simulink model "AGTF30SysSS_PExPIn"  (R2021b)
settings: Solver=FixedStepDiscrete  StartTime=0.0  StopTime=0; %MWS.In.Ts  FixedStep=1  RelTol=1e-3  EnableMultiTasking=on
values from neighbouring files (symbols this model uses):
  MWS = setup_initialize(MWS,startPt,SSsolverSP)    [Setup_Simulation.m]    (also in run_AGTF30e_script.m = Setup_Simulation(inputMethod,MWS.In,filename,Mdl,SSsolverSP,)
libraries: simulink x66, Lib_Solve_SSNRSolverJC_TMATS x1
(part 1 of 2)
settings Model: Creator=jwchapm2  LastModifiedBy=jlkratz
settings SolverCC: AlgebraicLoopSolver=TrustRegion
settings DataIOCC: LimitDataPoints=on  SaveFormat=Array  ReturnWorkspaceOutputs=off
settings OptimizationCC: LifeSpan=inf
settings DebuggingCC: SFUnexpectedBacktrackingDiag=warning  SFNoUnconditionalDefaultTransitionDiag=warning  SFExecutionAtInitializationDiag=none  SFMachineParentedDataDiag=warning  ArithmeticOperatorsInVariantConditions=warning
settings HardwareCC: ProdBitPerPointer=32  ProdBitPerSizeT=32  ProdBitPerPtrDiffT=32  ProdLargestAtomicFloat=None  ProdIntDivRoundTo=Undefined  ProdEndianess=Unspecified  ProdWordSize=32  ProdHWDeviceType=32-bit Generic
settings ModelReferenceCC: PropagateSignalLabelsOutOfModel=off
settings SFSimCC: SimUseLocalCustomCode=off  CustomCodeUndefinedFunction=UseInterfaceOnly
settings RTWCC: RTWUseLocalCustomCode=off
settings CodeAppCC: StateflowObjectComments=on
settings GRTTargetCC: TargetLangStandard=C89/C90 (ANSI)
settings ConfigComp: CovMetricSettings=dw  CovSaveCumulativeToWorkspaceVar=on  CovSaveSingleToWorkspaceVar=on  CovExternalEMLEnable=off

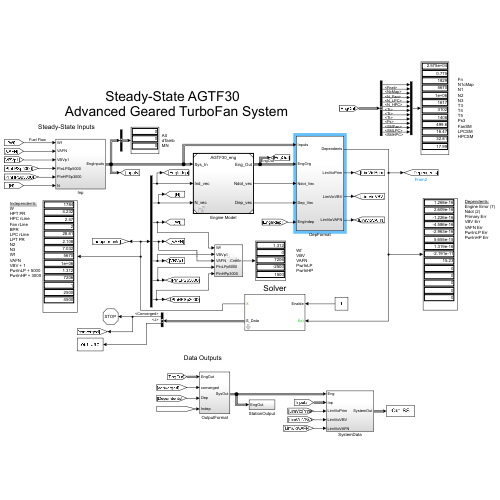
[thumbnail: Simulink's stored preview of the top-level diagram]
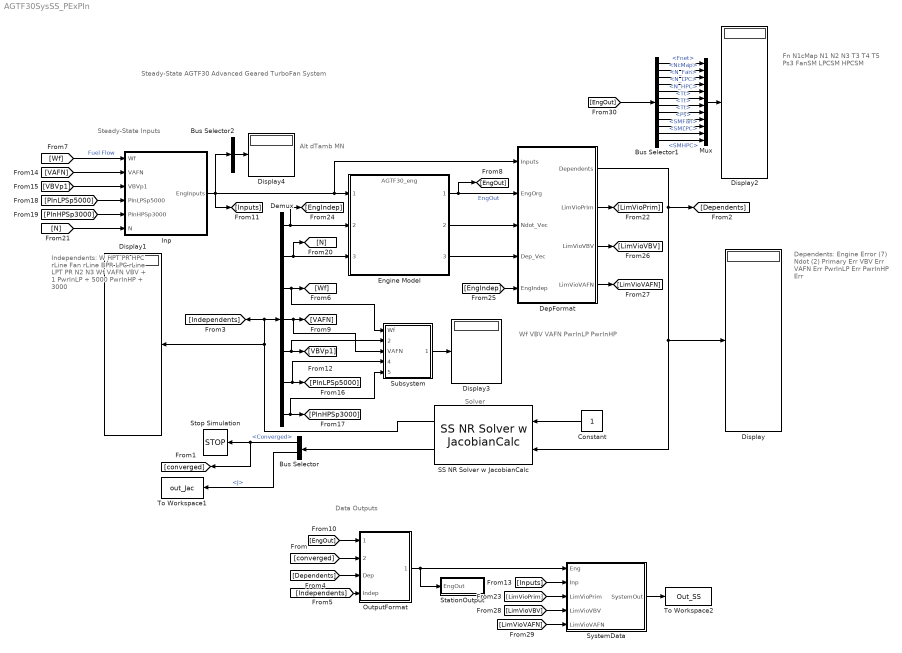
== system AGTF30SysSS_PExPIn ==
  note: Independents:
      | W
      | HPT PR
      | HPC rLine
      | Fan rLine
      | BPR
      | LPC rLine
      | LPT PR
      | N2
      | N3
      | Wf
      | VAFN
      | VBV + 1
      | PwrInLP + 5000
      | PwrInHP + 3000
  note: Dependents:
      | Engine Error (7)
      | Ndot (2)
      | Primary Err
      | VBV Err
      | VAFN Err
      | PwrInLP Err
      | PwrInHP Err
  note: Alt
      | dTamb
      | MN
  note: Wf
      | VBV
      | VAFN
      | PwrInLP
      | PwrInHP
  note: Fn
      | N1cMap
      | N1
      | N2
      | N3
      | T3
      | T4
      | T5
      | Ps3
      | FanSM
      | LPCSM
      | HPCSM
  note: Solver
  note: Steady-State Inputs
  note: Data Outputs
  note: Steady-State AGTF30
      | Advanced Geared TurboFan System
  Bus Selector : BusSelector  OutputSignals=Converged,J
  Bus Selector1 : BusSelector  OutputSignals=Perf.Fnet,Data.FAN_Data.NcMap,Shaft.N_Fan,Shaft.N_LPC,Shaft.N_HPC,S36.Tt,S4.Tt,S5.Tt,S36.Ps,SM.SMFan,SM.SMLPC,SM.SMHPC
  Bus Selector2 : BusSelector  OutputSignals=Altitude,dTamb,MN  OutputAsBus=on
  Constant : Constant
  Demux : Demux  Outputs=[7 2 1 1 1 1 1]
  DepFormat : Subsystem
  Display{,1..4} (5 alike) : Display
  Engine Model : ModelReference  ModelNameDialog=AGTF30_eng.mdl  SimulationMode=Normal  ModelReferenceVersion=14.20
  Inp : Subsystem
  Mux : Mux  Inputs=12
  OutputFormat : Subsystem
  SS NR Solver w JacobianCalc : Lib_Solve_SSNRSolverJC_TMATS/SS NR Solver w JacobianCalc  SJac_Per_M=MWS.Init.Solver.SS.JPer  SNR_IC_M=MWS.Init.Solver.SS.IC  SNR_DX_M=MWS.Init.Solver.SS.dX  SNR_Mx_M=1000000  SNR_Mn_M=0.000001  SJacobianAttempts_M=MWS.Init.Solver.SS.NRA  Cond_Limits_M=MWS.Init.Solver.SS.Lim
  StationOutput : Subsystem
  Stop Simulation : Stop
  Subsystem : Subsystem
  SystemData : Subsystem
  To Workspace1 : ToWorkspace  VariableName=out_Jac  SaveFormat=Timeseries  SampleTime=-1
      settings: MaxDataPoints=1
  To Workspace2 : ToWorkspace  VariableName=Out_SS  SaveFormat=Timeseries  SampleTime=-1
      settings: MaxDataPoints=1
  wires:
  Demux/2 -> [N], Engine Model/3
  Demux/1 -> [EngIndep], Engine Model/2
  Constant/1 -> SS NR Solver w JacobianCalc/1
  SS NR Solver w JacobianCalc/2 -> Bus Selector/1
  Bus Selector/1 -> Stop Simulation/1, [converged]  "<Converged>"
  Engine Model/1 -> [EngOut], DepFormat/2(EngOrg)  "EngOut"
  SS NR Solver w JacobianCalc/1 -> Display1/1, [Independents], Demux/1
  Demux/3 -> Subsystem/1(Wf), [Wf]
  DepFormat/1(Dependents) -> SS NR Solver w JacobianCalc/2, Display/1, [Dependents]
  Engine Model/2 -> DepFormat/3(Ndot_Vec)
  [converged] -> OutputFormat/2(converged)
  [Dependents] -> OutputFormat/3(Dep)
  [Independents] -> OutputFormat/4(Indep)
  [EngOut] -> OutputFormat/1(EngOut)
  Inp/1(EngInputs) -> Bus Selector2/1, [Inputs], DepFormat/1(Inputs), Engine Model/1
  [Wf] -> Inp/1(Wf)  "Fuel Flow"
  OutputFormat/1(SysOut) -> StationOutput/1(EngOut), SystemData/1(Eng)
  SystemData/1(SystemOut) -> To Workspace2/1
  [Inputs] -> SystemData/2(Inp)
  Engine Model/3 -> DepFormat/4(Dep_Vec)
  [VAFN] -> Inp/2(VAFN)
  Demux/4 -> Subsystem/3(VAFN), [VAFN]
  [VBVp1] -> Inp/3(VBVp1)
  Demux/6 -> Subsystem/4(PInLPp5000), [PInLPSp5000]
  Demux/7 -> [PInHPSp3000], Subsystem/5(PInHPp3000)
  [PInHPSp3000] -> Inp/5(PInHPSp3000)
  [PInLPSp5000] -> Inp/4(PInLPSp5000)
  [N] -> Inp/6(N)
  DepFormat/2(LimVioPrim) -> [LimVioPrim]
  [LimVioPrim] -> SystemData/3(LimVioPrim)
  [EngIndep] -> DepFormat/5(EngIndep)
  DepFormat/3(LimVioVBV) -> [LimVioVBV]
  DepFormat/4(LimVioVAFN) -> [LimVioVAFN]
  [LimVioVBV] -> SystemData/4(LimVioVBV)
  [LimVioVAFN] -> SystemData/5(LimVioVAFN)
  [EngOut] -> Bus Selector1/1
  Mux/1 -> Display2/1
  Subsystem/1(CntrlIn) -> Display3/1
  Demux/5 -> [VBVp1], Subsystem/2(VBVp1)
  Bus Selector2/1 -> Display4/1
  Bus Selector1/1 -> Mux/1  "<Fnet>"
  Bus Selector1/3 -> Mux/3  "<N_Fan>"
  Bus Selector1/5 -> Mux/5  "<N_HPC>"
  Bus Selector1/4 -> Mux/4  "<N_LPC>"
  Bus Selector1/6 -> Mux/6  "<Tt>"
  Bus Selector1/7 -> Mux/7  "<Tt>"
  Bus Selector1/8 -> Mux/8  "<Tt>"
  Bus Selector1/10 -> Mux/10  "<SMFan>"
  Bus Selector1/9 -> Mux/9  "<Ps>"
  Bus Selector1/11 -> Mux/11  "<SMLPC>"
  Bus Selector1/12 -> Mux/12  "<SMHPC>"
  Bus Selector/2 -> To Workspace1/1  "<J>"
  Bus Selector1/2 -> Mux/2  "<NcMap>"

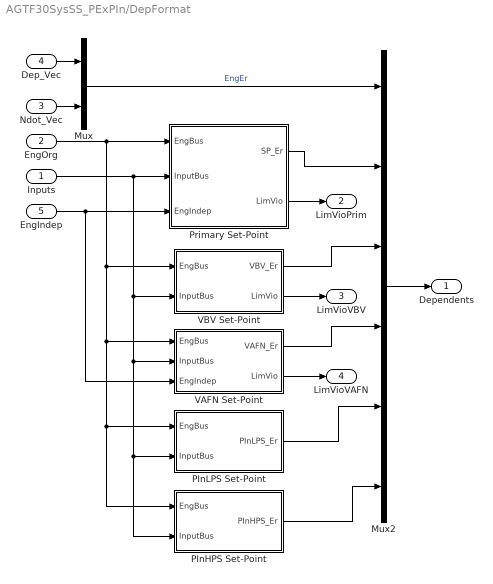
== system AGTF30SysSS_PExPIn/DepFormat ==
  Inputs : Inport
  EngOrg : Inport  Port=2
  Ndot_Vec : Inport  Port=3
  Dep_Vec : Inport  Port=4
  EngIndep : Inport  Port=5
  Mux : Mux  Inputs=2
  Mux2 : Mux  Inputs=6
  PInHPS Set-Point : Subsystem
  PInLPS Set-Point : Subsystem
  Primary Set-Point : Subsystem
  VAFN Set-Point : Subsystem
  VBV Set-Point : Subsystem
  Dependents : Outport
  LimVioPrim : Outport  Port=2
  LimVioVBV : Outport  Port=3
  LimVioVAFN : Outport  Port=4
  wires:
  Ndot_Vec/1 -> Mux/2
  Mux/1 -> Mux2/1  "EngEr"
  Mux2/1 -> Dependents/1
  Dep_Vec/1 -> Mux/1
  EngOrg/1 -> PInHPS Set-Point/1(EngBus), PInLPS Set-Point/1(EngBus), VAFN Set-Point/1(EngBus), VBV Set-Point/1(EngBus), Primary Set-Point/1(EngBus)
  Inputs/1 -> Primary Set-Point/2(InputBus), PInHPS Set-Point/2(InputBus), PInLPS Set-Point/2(InputBus), VAFN Set-Point/2(InputBus), VBV Set-Point/2(InputBus)
  Primary Set-Point/1(SP_Er) -> Mux2/2
  VBV Set-Point/1(VBV_Er) -> Mux2/3
  VAFN Set-Point/1(VAFN_Er) -> Mux2/4
  PInLPS Set-Point/1(PInLPS_Er) -> Mux2/5
  PInHPS Set-Point/1(PInHPS_Er) -> Mux2/6
  Primary Set-Point/2(LimVio) -> LimVioPrim/1
  EngIndep/1 -> VAFN Set-Point/3(EngIndep), Primary Set-Point/3(EngIndep)
  VAFN Set-Point/2(LimVio) -> LimVioVAFN/1
  VBV Set-Point/2(LimVio) -> LimVioVBV/1

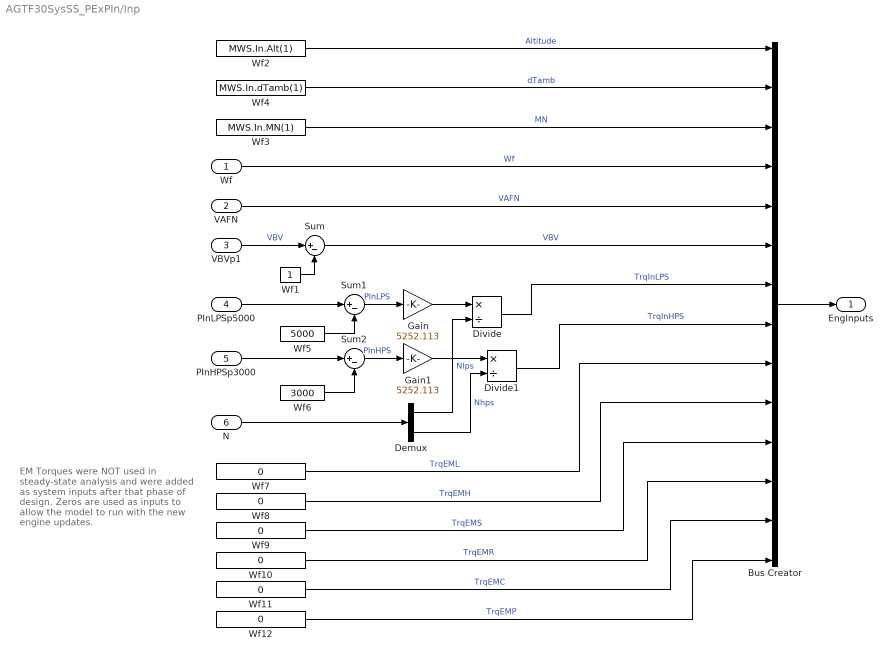
== system AGTF30SysSS_PExPIn/Inp ==
  note: EM Torques were NOT used
      | in steady-state analysis and were
      | added as system inputs after that
      | phase of design. Zeros are used as
      | inputs to allow the model to run with
      | the new engine updates.
  Wf : Inport
  VAFN : Inport  Port=2
  VBVp1 : Inport  Port=3
  PInLPSp5000 : Inport  Port=4
  PInHPSp3000 : Inport  Port=5
  N : Inport  Port=6
  Bus Creator : BusCreator  Inputs=14
  Demux : Demux  Outputs=2
  Divide : Product  Inputs=*/
  Divide1 : Product  Inputs=*/
  Gain : Gain  Gain=5252.113
  Gain1 : Gain  Gain=5252.113
  Sum : Sum  Inputs=|+-
  Sum1 : Sum  Inputs=|+-
  Sum2 : Sum  Inputs=|+-
  Wf1 : Constant
  Wf{7..12} (6 alike) : Constant  Value=0
  Wf2 : Constant  Value=MWS.In.Alt(1)
  Wf3 : Constant  Value=MWS.In.MN(1)
  Wf4 : Constant  Value=MWS.In.dTamb(1)
  Wf5 : Constant  Value=5000
  Wf6 : Constant  Value=3000
  EngInputs : Outport
  wires:
  Wf2/1 -> Bus Creator/1  "Altitude"
  Wf3/1 -> Bus Creator/3  "MN"
  Bus Creator/1 -> EngInputs/1
  Sum/1 -> Bus Creator/6  "VBV"
  VAFN/1 -> Bus Creator/5  "VAFN"
  Wf4/1 -> Bus Creator/2  "dTamb"
  Wf/1 -> Bus Creator/4  "Wf"
  VBVp1/1 -> Sum/1  "VBV"
  Wf1/1 -> Sum/2
  PInLPSp5000/1 -> Sum1/1
  Wf5/1 -> Sum1/2
  PInHPSp3000/1 -> Sum2/1
  Wf6/1 -> Sum2/2
  Divide/1 -> Bus Creator/7  "TrqInLPS"
  Divide1/1 -> Bus Creator/8  "TrqInHPS"
  N/1 -> Demux/1
  Sum1/1 -> Gain/1  "PInLPS"
  Sum2/1 -> Gain1/1  "PInHPS"
  Gain/1 -> Divide/1
  Gain1/1 -> Divide1/1
  Demux/1 -> Divide/2  "Nlps"
  Demux/2 -> Divide1/2  "Nhps"
  Wf7/1 -> Bus Creator/9  "TrqEML"
  Wf8/1 -> Bus Creator/10  "TrqEMH"
  Wf9/1 -> Bus Creator/11  "TrqEMS"
  Wf10/1 -> Bus Creator/12  "TrqEMR"
  Wf11/1 -> Bus Creator/13  "TrqEMC"
  Wf12/1 -> Bus Creator/14  "TrqEMP"

== system AGTF30SysSS_PExPIn/OutputFormat ==
  EngOut : Inport
  converged : Inport  Port=2
  Dep : Inport  Port=3
  Indep : Inport  Port=4
  Bus Creator : BusCreator  Inputs=3
  Bus Creator1 : BusCreator  Inputs=2
  Signal Conversion : SignalConversion  OverrideOpt=off
  Signal Conversion1 : SignalConversion  OverrideOpt=off
  Signal Conversion2 : SignalConversion  OverrideOpt=off
  SysOut : Outport
  wires:
  Signal Conversion1/1 -> Bus Creator/2  "dependents"
  Signal Conversion/1 -> Bus Creator/3  "independents"
  Signal Conversion2/1 -> Bus Creator/1  "converged"
  Bus Creator1/1 -> SysOut/1  "SysOut"
  Bus Creator/1 -> Bus Creator1/2  "Solver"
  Indep/1 -> Signal Conversion/1
  Dep/1 -> Signal Conversion1/1
  converged/1 -> Signal Conversion2/1
  EngOut/1 -> Bus Creator1/1  "EngOut"

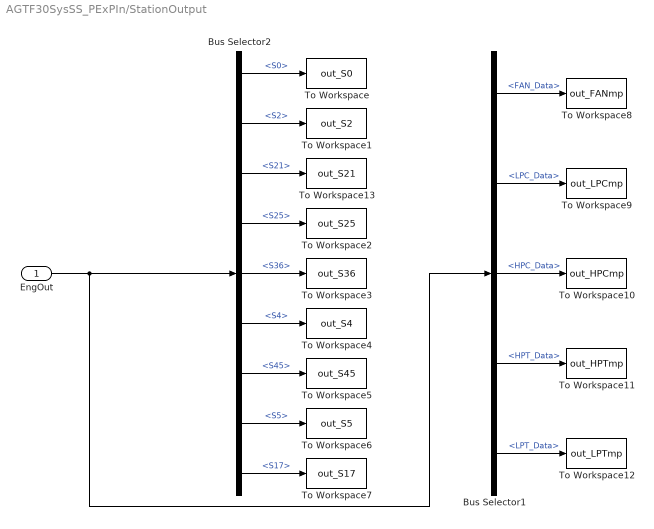
== system AGTF30SysSS_PExPIn/StationOutput ==
  EngOut : Inport
  Bus Selector1 : BusSelector  OutputSignals=EngOut.Data.FAN_Data,EngOut.Data.LPC_Data,EngOut.Data.HPC_Data,EngOut.Data.HPT_Data,EngOut.Data.LPT_Data
  Bus Selector2 : BusSelector  OutputSignals=EngOut.S0,EngOut.S2,EngOut.S21,EngOut.S25,EngOut.S36,EngOut.S4,EngOut.S45,EngOut.S5,EngOut.S17
  To Workspace : ToWorkspace  VariableName=out_S0  SaveFormat=Timeseries  SampleTime=-1
  To Workspace1 : ToWorkspace  VariableName=out_S2  SaveFormat=Timeseries  SampleTime=-1
  To Workspace10 : ToWorkspace  VariableName=out_HPCmp  SaveFormat=Timeseries  SampleTime=-1
  To Workspace11 : ToWorkspace  VariableName=out_HPTmp  SaveFormat=Timeseries  SampleTime=-1
  To Workspace12 : ToWorkspace  VariableName=out_LPTmp  SaveFormat=Timeseries  SampleTime=-1
  To Workspace13 : ToWorkspace  VariableName=out_S21  SaveFormat=Timeseries  SampleTime=-1
  To Workspace2 : ToWorkspace  VariableName=out_S25  SaveFormat=Timeseries  SampleTime=-1
  To Workspace3 : ToWorkspace  VariableName=out_S36  SaveFormat=Timeseries  SampleTime=-1
  To Workspace4 : ToWorkspace  VariableName=out_S4  SaveFormat=Timeseries  SampleTime=-1
  To Workspace5 : ToWorkspace  VariableName=out_S45  SaveFormat=Timeseries  SampleTime=-1
  To Workspace6 : ToWorkspace  VariableName=out_S5  SaveFormat=Timeseries  SampleTime=-1
  To Workspace7 : ToWorkspace  VariableName=out_S17  SaveFormat=Timeseries  SampleTime=-1
  To Workspace8 : ToWorkspace  VariableName=out_FANmp  SaveFormat=Timeseries  SampleTime=-1
  To Workspace9 : ToWorkspace  VariableName=out_LPCmp  SaveFormat=Timeseries  SampleTime=-1
  wires:
  Bus Selector1/5 -> To Workspace12/1  "<LPT_Data>"
  Bus Selector1/4 -> To Workspace11/1  "<HPT_Data>"
  Bus Selector1/3 -> To Workspace10/1  "<HPC_Data>"
  Bus Selector1/2 -> To Workspace9/1  "<LPC_Data>"
  Bus Selector1/1 -> To Workspace8/1  "<FAN_Data>"
  Bus Selector2/9 -> To Workspace7/1  "<S17>"
  Bus Selector2/8 -> To Workspace6/1  "<S5>"
  Bus Selector2/7 -> To Workspace5/1  "<S45>"
  Bus Selector2/6 -> To Workspace4/1  "<S4>"
  Bus Selector2/5 -> To Workspace3/1  "<S36>"
  Bus Selector2/4 -> To Workspace2/1  "<S25>"
  Bus Selector2/2 -> To Workspace1/1  "<S2>"
  EngOut/1 -> Bus Selector2/1, Bus Selector1/1
  Bus Selector2/1 -> To Workspace/1  "<S0>"
  Bus Selector2/3 -> To Workspace13/1  "<S21>"

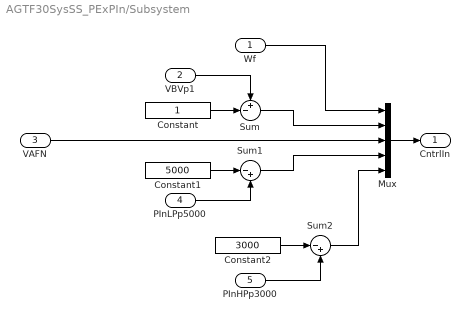
== system AGTF30SysSS_PExPIn/Subsystem ==
  Wf : Inport
  VBVp1 : Inport  Port=2
  VAFN : Inport  Port=3
  PInLPp5000 : Inport  Port=4
  PInHPp3000 : Inport  Port=5
  Constant : Constant
  Constant1 : Constant  Value=5000
  Constant2 : Constant  Value=3000
  Mux : Mux  Inputs=5
  Sum : Sum  Inputs=+-|
  Sum1 : Sum  Inputs=|-+
  Sum2 : Sum  Inputs=|-+
  CntrlIn : Outport
  wires:
  Mux/1 -> CntrlIn/1
  VAFN/1 -> Mux/3
  VBVp1/1 -> Sum/1
  Wf/1 -> Mux/1
  PInLPp5000/1 -> Sum1/2
  Constant/1 -> Sum/2
  Sum/1 -> Mux/2
  Constant1/1 -> Sum1/1
  Sum1/1 -> Mux/4
  PInHPp3000/1 -> Sum2/2
  Constant2/1 -> Sum2/1
  Sum2/1 -> Mux/5

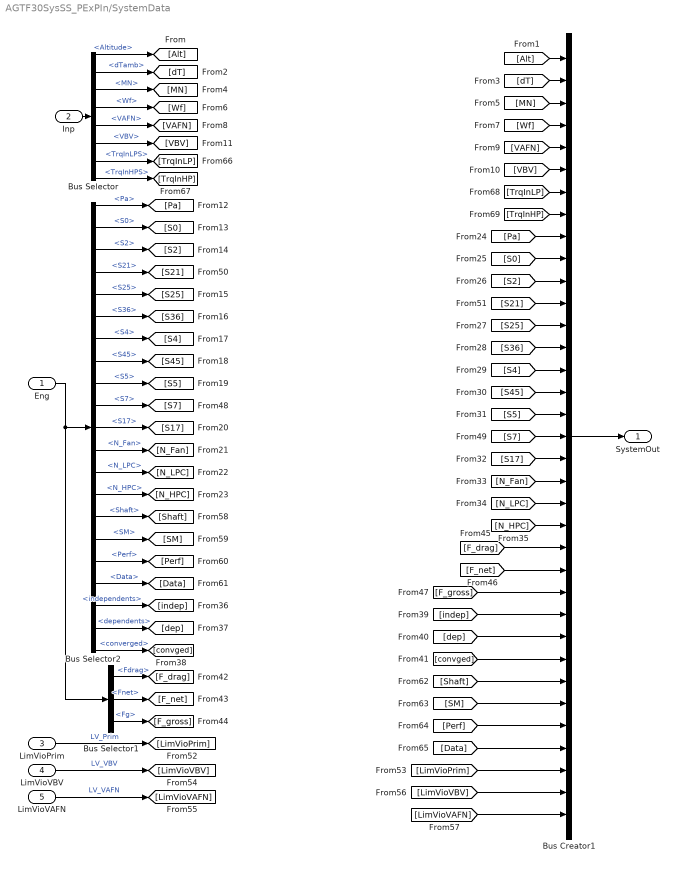
== system AGTF30SysSS_PExPIn/SystemData ==
  Eng : Inport
  Inp : Inport  Port=2
  LimVioPrim : Inport  Port=3
  LimVioVBV : Inport  Port=4
  LimVioVAFN : Inport  Port=5
  Bus Creator1 : BusCreator  Inputs=35
  Bus Selector : BusSelector  OutputSignals=Altitude,dTamb,MN,Wf,VAFN,VBV,TrqInLPS,TrqInHPS
  Bus Selector1 : BusSelector  OutputSignals=EngOut.Perf.Fdrag,EngOut.Perf.Fnet,EngOut.Perf.Fg
  Bus Selector2 : BusSelector  OutputSignals=EngOut.Amb.Pa,EngOut.S0,EngOut.S2,EngOut.S21,EngOut.S25,EngOut.S36,EngOut.S4,EngOut.S45,EngOut.S5,EngOut.S7,EngOut.S17,EngOut.Shaft.N_Fan,EngOut.Shaft.N_LPC,EngOut.Shaft.N_HPC,EngOut.Shaft,EngOut.SM,EngOut.Perf,EngOut.Data,Solver.independents,Solver.dependents,Solver.converged
  SystemOut : Outport
  wires:
  Eng/1 -> Bus Selector1/1, Bus Selector2/1
  Bus Creator1/1 -> SystemOut/1
  Inp/1 -> Bus Selector/1
  [S2] -> Bus Creator1/11
  [S0] -> Bus Creator1/10
  [Pa] -> Bus Creator1/9
  Bus Selector/6 -> [VBV]  "<VBV>"
  Bus Selector/4 -> [Wf]  "<Wf>"
  Bus Selector/3 -> [MN]  "<MN>"
  Bus Selector/1 -> [Alt]  "<Altitude>"
  [Alt] -> Bus Creator1/1
  [dT] -> Bus Creator1/2
  [MN] -> Bus Creator1/3
  [Wf] -> Bus Creator1/4
  [VAFN] -> Bus Creator1/5
  [VBV] -> Bus Creator1/6
  Bus Selector2/1 -> [Pa]  "<Pa>"
  Bus Selector2/2 -> [S0]  "<S0>"
  Bus Selector2/3 -> [S2]  "<S2>"
  Bus Selector2/5 -> [S25]  "<S25>"
  Bus Selector2/6 -> [S36]  "<S36>"
  Bus Selector2/7 -> [S4]  "<S4>"
  Bus Selector2/8 -> [S45]  "<S45>"
  Bus Selector2/9 -> [S5]  "<S5>"
  Bus Selector2/11 -> [S17]  "<S17>"
  Bus Selector2/12 -> [N_Fan]  "<N_Fan>"
  Bus Selector2/13 -> [N_LPC]  "<N_LPC>"
  Bus Selector2/14 -> [N_HPC]  "<N_HPC>"
  Bus Selector2/19 -> [indep]  "<independents>"
  Bus Selector2/20 -> [dep]  "<dependents>"
  Bus Selector2/21 -> [convged]  "<converged>"
  Bus Selector1/1 -> [F_drag]  "<Fdrag>"
  Bus Selector1/2 -> [F_net]  "<Fnet>"
  Bus Selector1/3 -> [F_gross]  "<Fg>"
  Bus Selector2/10 -> [S7]  "<S7>"
  Bus Selector2/4 -> [S21]  "<S21>"
  [S21] -> Bus Creator1/12
  [S4] -> Bus Creator1/15
  [S45] -> Bus Creator1/16
  [S17] -> Bus Creator1/19
  [S5] -> Bus Creator1/17
  [N_Fan] -> Bus Creator1/20
  [S25] -> Bus Creator1/13
  [S36] -> Bus Creator1/14
  [S7] -> Bus Creator1/18
  [N_LPC] -> Bus Creator1/21
  [N_HPC] -> Bus Creator1/22
  [F_drag] -> Bus Creator1/23
  [F_net] -> Bus Creator1/24
  [F_gross] -> Bus Creator1/25
  [convged] -> Bus Creator1/28
  [indep] -> Bus Creator1/26
  [dep] -> Bus Creator1/27
  LimVioPrim/1 -> [LimVioPrim]  "LV_Prim"
  [LimVioPrim] -> Bus Creator1/33
  LimVioVBV/1 -> [LimVioVBV]  "LV_VBV"
  LimVioVAFN/1 -> [LimVioVAFN]  "LV_VAFN"
  [LimVioVBV] -> Bus Creator1/34
  [LimVioVAFN] -> Bus Creator1/35
  Bus Selector2/15 -> [Shaft]  "<Shaft>"
  Bus Selector2/16 -> [SM]  "<SM>"
  Bus Selector2/17 -> [Perf]  "<Perf>"
  Bus Selector2/18 -> [Data]  "<Data>"
  [Shaft] -> Bus Creator1/29
  [SM] -> Bus Creator1/30
  [Perf] -> Bus Creator1/31
  [Data] -> Bus Creator1/32
  Bus Selector/2 -> [dT]  "<dTamb>"
  Bus Selector/5 -> [VAFN]  "<VAFN>"
  Bus Selector/7 -> [TrqInLP]  "<TrqInLPS>"
  Bus Selector/8 -> [TrqInHP]  "<TrqInHPS>"
  [TrqInHP] -> Bus Creator1/8
  [TrqInLP] -> Bus Creator1/7

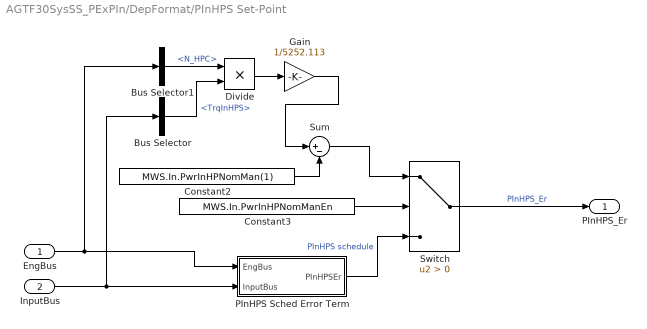
== system AGTF30SysSS_PExPIn/DepFormat/PInHPS Set-Point ==
  EngBus : Inport
  InputBus : Inport  Port=2
  Bus Selector : BusSelector  OutputSignals=TrqInHPS
  Bus Selector1 : BusSelector  OutputSignals=Shaft.N_HPC
  Constant2 : Constant  Value=MWS.In.PwrInHPNomMan(1)
  Constant3 : Constant  Value=MWS.In.PwrInHPNomManEn
  Divide : Product  Inputs=**
  Gain : Gain  Gain=1/5252.113
  PInHPS Sched Error Term : Subsystem
  Sum : Sum  Inputs=|+-
  Switch : Switch  Criteria=u2 > Threshold
  PInHPS_Er : Outport
  wires:
  PInHPS Sched Error Term/1(PInHPSEr) -> Switch/3  "PInHPS schedule"
  Constant3/1 -> Switch/2
  Constant2/1 -> Sum/2
  Switch/1 -> PInHPS_Er/1  "PInHPS_Er"
  Gain/1 -> Sum/1
  Bus Selector/1 -> Divide/2  "<TrqInHPS>"
  Sum/1 -> Switch/1
  Divide/1 -> Gain/1
  EngBus/1 -> Bus Selector1/1, PInHPS Sched Error Term/1(EngBus)
  Bus Selector1/1 -> Divide/1  "<N_HPC>"
  InputBus/1 -> PInHPS Sched Error Term/2(InputBus), Bus Selector/1

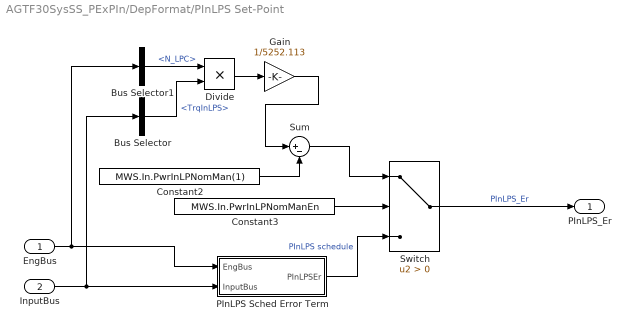
== system AGTF30SysSS_PExPIn/DepFormat/PInLPS Set-Point ==
  EngBus : Inport
  InputBus : Inport  Port=2
  Bus Selector : BusSelector  OutputSignals=TrqInLPS
  Bus Selector1 : BusSelector  OutputSignals=Shaft.N_LPC
  Constant2 : Constant  Value=MWS.In.PwrInLPNomMan(1)
  Constant3 : Constant  Value=MWS.In.PwrInLPNomManEn
  Divide : Product  Inputs=**
  Gain : Gain  Gain=1/5252.113
  PInLPS Sched Error Term : Subsystem
  Sum : Sum  Inputs=|+-
  Switch : Switch  Criteria=u2 > Threshold
  PInLPS_Er : Outport
  wires:
  Switch/1 -> PInLPS_Er/1  "PInLPS_Er"
  Constant3/1 -> Switch/2
  InputBus/1 -> Bus Selector/1, PInLPS Sched Error Term/2(InputBus)
  EngBus/1 -> Bus Selector1/1, PInLPS Sched Error Term/1(EngBus)
  PInLPS Sched Error Term/1(PInLPSEr) -> Switch/3  "PInLPS schedule"
  Constant2/1 -> Sum/2
  Sum/1 -> Switch/1
  Bus Selector1/1 -> Divide/1  "<N_LPC>"
  Bus Selector/1 -> Divide/2  "<TrqInLPS>"
  Divide/1 -> Gain/1
  Gain/1 -> Sum/1

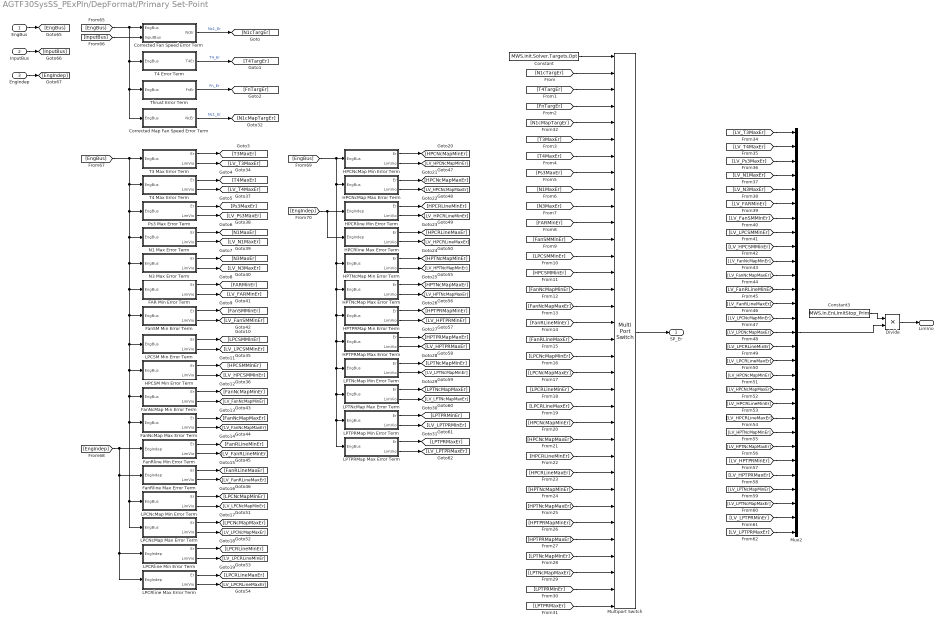
== system AGTF30SysSS_PExPIn/DepFormat/Primary Set-Point ==
  EngBus : Inport
  InputBus : Inport  Port=2
  EngIndep : Inport  Port=3
  Constant : Constant  Value=MWS.Init.Solver.Targets.Opt
  Constant3 : Constant  Value=MWS.In.EnLimitStop_Prim
  Corrected Fan Speed Error Term : Subsystem
  Corrected Map Fan Speed Error Term : Subsystem
  Divide : Product  Inputs=**
  FAR Min Error Term : Subsystem
  FanNcMap Max Error Term : Subsystem
  FanNcMap Min Error Term : Subsystem
  FanRline Max Error Term : Subsystem
  FanRline Min Error Term : Subsystem
  FanSM Min Error Term : Subsystem
  HPCNcMap Max Error Term : Subsystem
  HPCNcMap Min Error Term : Subsystem
  HPCRline Max Error Term : Subsystem
  HPCRline Min Error Term : Subsystem
  HPCSM Min Error Term : Subsystem
  HPTNcMap Max Error Term : Subsystem
  HPTNcMap Min Error Term : Subsystem
  HPTPRMap Max Error Term : Subsystem
  HPTPRMap Min Error Term : Subsystem
  LPCNcMap Max Error Term : Subsystem
  LPCNcMap Min Error Term : Subsystem
  LPCRline Max Error Term : Subsystem
  LPCRline Min Error Term : Subsystem
  LPCSM Min Error Term : Subsystem
  LPTNcMap Max Error Term : Subsystem
  LPTNcMap Min Error Term : Subsystem
  LPTPRMap Max Error Term : Subsystem
  LPTPRMap Min Error Term : Subsystem
  Multiport Switch : MultiPortSwitch  Inputs=33
  Mux2 : Mux  Inputs=29
  N1 Max Error Term : Subsystem
  N3 Max Error Term : Subsystem
  Ps3 Max Error Term : Subsystem
  T3 Max Error Term : Subsystem
  T4 Error Term : Subsystem
  T4 Max Error Term : Subsystem
  Thrust Error Term : Subsystem
  SP_Er : Outport
  LimVio : Outport  Port=2
  wires:
  Corrected Fan Speed Error Term/1(NcEr) -> [N1cTargEr]  "Nc1_Er"
  [N1cTargEr] -> Multiport Switch/2
  [T4TargEr] -> Multiport Switch/3
  [FnTargEr] -> Multiport Switch/4
  [LPTPRMaxEr] -> Multiport Switch/34
  [LPTPRMinEr] -> Multiport Switch/33
  [LPTNcMapMaxEr] -> Multiport Switch/32
  [LPTNcMapMinEr] -> Multiport Switch/31
  [HPTPRMapMaxEr] -> Multiport Switch/30
  [HPTPRMapMinEr] -> Multiport Switch/29
  [HPTNcMapMaxEr] -> Multiport Switch/28
  [HPTNcMapMinEr] -> Multiport Switch/27
  [HPCRLineMaxEr] -> Multiport Switch/26
  [HPCRLineMinEr] -> Multiport Switch/25
  [HPCNcMapMaxEr] -> Multiport Switch/24
  [HPCNcMapMinEr] -> Multiport Switch/23
  [LPCRLineMaxEr] -> Multiport Switch/22
  [LPCRLineMinEr] -> Multiport Switch/21
  [LPCNcMapMaxEr] -> Multiport Switch/20
  [LPCNcMapMinEr] -> Multiport Switch/19
  [FanRLineMaxEr] -> Multiport Switch/18
  [FanRLineMinEr] -> Multiport Switch/17
  [FanNcMapMaxEr] -> Multiport Switch/16
  [FanNcMapMinEr] -> Multiport Switch/15
  [HPCSMMinEr] -> Multiport Switch/14
  [LPCSMMinEr] -> Multiport Switch/13
  [FanSMMinEr] -> Multiport Switch/12
  [FARMinEr] -> Multiport Switch/11
  [N3MaxEr] -> Multiport Switch/10
  [N1MaxEr] -> Multiport Switch/9
  [Ps3MaxEr] -> Multiport Switch/8
  [T4MaxEr] -> Multiport Switch/7
  [T3MaxEr] -> Multiport Switch/6
  Constant/1 -> Multiport Switch/1
  Multiport Switch/1 -> SP_Er/1
  Constant3/1 -> Divide/1
  [LV_T3MaxEr] -> Mux2/1
  [LV_T4MaxEr] -> Mux2/2
  [LV_Ps3MaxEr] -> Mux2/3
  [LV_N1MaxEr] -> Mux2/4
  [LV_N3MaxEr] -> Mux2/5
  [LV_FARMinEr] -> Mux2/6
  [LV_FanSMMinEr] -> Mux2/7
  [LV_LPCSMMinEr] -> Mux2/8
  [LV_HPCSMMinEr] -> Mux2/9
  [LV_FanNcMapMinEr] -> Mux2/10
  [LV_FanNcMapMaxEr] -> Mux2/11
  [LV_FanRLineMinEr] -> Mux2/12
  [LV_FanRLineMaxEr] -> Mux2/13
  [LV_LPCNcMapMinEr] -> Mux2/14
  [LV_LPCNcMapMaxEr] -> Mux2/15
  [LV_LPCRLineMinEr] -> Mux2/16
  [LV_LPCRLineMaxEr] -> Mux2/17
  [LV_HPCNcMapMinEr] -> Mux2/18
  [LV_HPCNcMapMaxEr] -> Mux2/19
  [LV_HPCRLineMinEr] -> Mux2/20
  [LV_HPCRLineMaxEr] -> Mux2/21
  [LV_HPTNcMapMinEr] -> Mux2/22
  [LV_HPTNcMapMaxEr] -> Mux2/23
  [LV_HPTPRMinEr] -> Mux2/24
  [LV_HPTPRMaxEr] -> Mux2/25
  [LV_LPTNcMapMinEr] -> Mux2/26
  [LV_LPTNcMapMaxEr] -> Mux2/27
  [LV_LPTPRMinEr] -> Mux2/28
  [LV_LPTPRMaxEr] -> Mux2/29
  Mux2/1 -> Divide/2
  Divide/1 -> LimVio/1
  EngBus/1 -> [EngBus]
  InputBus/1 -> [InputBus]
  [InputBus] -> Corrected Fan Speed Error Term/2(InputBus)
  [EngBus] -> Corrected Fan Speed Error Term/1(EngBus), T4 Error Term/1(EngBus), Corrected Map Fan Speed Error Term/1(EngBus), Thrust Error Term/1(EngBus)
  T4 Error Term/1(T4Er) -> [T4TargEr]  "T4_Er"
  Thrust Error Term/1(FnEr) -> [FnTargEr]  "Fn_Er"
  [EngBus] -> LPCNcMap Max Error Term/1(EngBus), LPCNcMap Min Error Term/1(EngBus), FanNcMap Max Error Term/1(EngBus), FanNcMap Min Error Term/1(EngBus), HPCSM Min Error Term/1(EngBus), LPCSM Min Error Term/1(EngBus), FanSM Min Error Term/1(EngBus), FAR Min Error Term/1(EngBus), N3 Max Error Term/1(EngBus), N1 Max Error Term/1(EngBus), Ps3 Max Error Term/1(EngBus), T4 Max Error Term/1(EngBus), T3 Max Error Term/1(EngBus)
  T3 Max Error Term/1(Er) -> [T3MaxEr]
  T3 Max Error Term/2(LimVio) -> [LV_T3MaxEr]
  T4 Max Error Term/1(Er) -> [T4MaxEr]
  T4 Max Error Term/2(LimVio) -> [LV_T4MaxEr]
  Ps3 Max Error Term/2(LimVio) -> [LV_Ps3MaxEr]
  Ps3 Max Error Term/1(Er) -> [Ps3MaxEr]
  N1 Max Error Term/1(Er) -> [N1MaxEr]
  N1 Max Error Term/2(LimVio) -> [LV_N1MaxEr]
  N3 Max Error Term/1(Er) -> [N3MaxEr]
  N3 Max Error Term/2(LimVio) -> [LV_N3MaxEr]
  FAR Min Error Term/2(LimVio) -> [LV_FARMinEr]
  FAR Min Error Term/1(Er) -> [FARMinEr]
  FanSM Min Error Term/2(LimVio) -> [LV_FanSMMinEr]
  FanSM Min Error Term/1(Er) -> [FanSMMinEr]
  LPCSM Min Error Term/1(Er) -> [LPCSMMinEr]
  LPCSM Min Error Term/2(LimVio) -> [LV_LPCSMMinEr]
  HPCSM Min Error Term/2(LimVio) -> [LV_HPCSMMinEr]
  HPCSM Min Error Term/1(Er) -> [HPCSMMinEr]
  FanNcMap Max Error Term/2(LimVio) -> [LV_FanNcMapMaxEr]
  FanNcMap Max Error Term/1(Er) -> [FanNcMapMaxEr]
  FanNcMap Min Error Term/2(LimVio) -> [LV_FanNcMapMinEr]
  FanNcMap Min Error Term/1(Er) -> [FanNcMapMinEr]
  EngIndep/1 -> [EngIndep]
  [EngIndep] -> LPCRline Max Error Term/1(EngIndep), LPCRline Min Error Term/1(EngIndep), FanRline Max Error Term/1(EngIndep), FanRline Min Error Term/1(EngIndep)
  FanRline Min Error Term/1(Er) -> [FanRLineMinEr]
  FanRline Min Error Term/2(LimVio) -> [LV_FanRLineMinEr]
  FanRline Max Error Term/1(Er) -> [FanRLineMaxEr]
  FanRline Max Error Term/2(LimVio) -> [LV_FanRLineMaxEr]
  LPCNcMap Min Error Term/1(Er) -> [LPCNcMapMinEr]
  LPCNcMap Min Error Term/2(LimVio) -> [LV_LPCNcMapMinEr]
  LPCNcMap Max Error Term/1(Er) -> [LPCNcMapMaxEr]
  LPCNcMap Max Error Term/2(LimVio) -> [LV_LPCNcMapMaxEr]
  LPCRline Min Error Term/1(Er) -> [LPCRLineMinEr]
  LPCRline Min Error Term/2(LimVio) -> [LV_LPCRLineMinEr]
  LPCRline Max Error Term/1(Er) -> [LPCRLineMaxEr]
  LPCRline Max Error Term/2(LimVio) -> [LV_LPCRLineMaxEr]
  [EngBus] -> LPTPRMap Max Error Term/1(EngBus), LPTPRMap Min Error Term/1(EngBus), LPTNcMap Max Error Term/1(EngBus), LPTNcMap Min Error Term/1(EngBus), HPTPRMap Max Error Term/1(EngBus), HPTPRMap Min Error Term/1(EngBus), HPTNcMap Max Error Term/1(EngBus), HPTNcMap Min Error Term/1(EngBus), HPCNcMap Max Error Term/1(EngBus), HPCNcMap Min Error Term/1(EngBus)
  HPCNcMap Min Error Term/1(Er) -> [HPCNcMapMinEr]
  HPCNcMap Min Error Term/2(LimVio) -> [LV_HPCNcMapMinEr]
  HPCNcMap Max Error Term/1(Er) -> [HPCNcMapMaxEr]
  HPCNcMap Max Error Term/2(LimVio) -> [LV_HPCNcMapMaxEr]
  HPCRline Min Error Term/1(Er) -> [HPCRLineMinEr]
  HPCRline Min Error Term/2(LimVio) -> [LV_HPCRLineMinEr]
  HPCRline Max Error Term/1(Er) -> [HPCRLineMaxEr]
  HPCRline Max Error Term/2(LimVio) -> [LV_HPCRLineMaxEr]
  [EngIndep] -> HPCRline Max Error Term/1(EngIndep), HPCRline Min Error Term/1(EngIndep)
  HPTNcMap Min Error Term/1(Er) -> [HPTNcMapMinEr]
  HPTNcMap Min Error Term/2(LimVio) -> [LV_HPTNcMapMinEr]
  HPTNcMap Max Error Term/1(Er) -> [HPTNcMapMaxEr]
  HPTNcMap Max Error Term/2(LimVio) -> [LV_HPTNcMapMaxEr]
  HPTPRMap Min Error Term/2(LimVio) -> [LV_HPTPRMinEr]
  HPTPRMap Min Error Term/1(Er) -> [HPTPRMapMinEr]
  HPTPRMap Max Error Term/1(Er) -> [HPTPRMapMaxEr]
  HPTPRMap Max Error Term/2(LimVio) -> [LV_HPTPRMaxEr]
  LPTNcMap Min Error Term/2(LimVio) -> [LV_LPTNcMapMinEr]
  LPTNcMap Min Error Term/1(Er) -> [LPTNcMapMinEr]
  LPTNcMap Max Error Term/2(LimVio) -> [LV_LPTNcMapMaxEr]
  LPTNcMap Max Error Term/1(Er) -> [LPTNcMapMaxEr]
  LPTPRMap Min Error Term/1(Er) -> [LPTPRMinEr]
  LPTPRMap Min Error Term/2(LimVio) -> [LV_LPTPRMinEr]
  LPTPRMap Max Error Term/1(Er) -> [LPTPRMaxEr]
  LPTPRMap Max Error Term/2(LimVio) -> [LV_LPTPRMaxEr]
  Corrected Map Fan Speed Error Term/1(NcEr) -> [N1cMapTargEr]  "Nc1_Er"
  [N1cMapTargEr] -> Multiport Switch/5

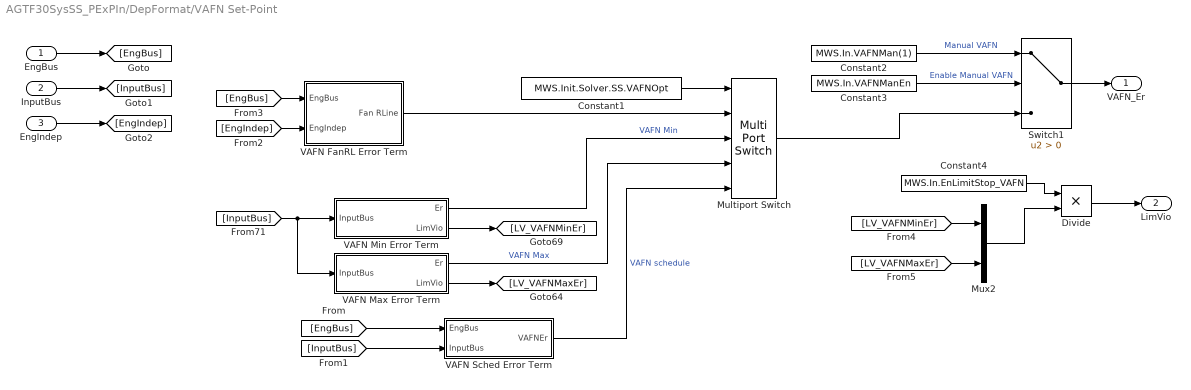
== system AGTF30SysSS_PExPIn/DepFormat/VAFN Set-Point ==
  EngBus : Inport
  InputBus : Inport  Port=2
  EngIndep : Inport  Port=3
  Constant1 : Constant  Value=MWS.Init.Solver.SS.VAFNOpt
  Constant2 : Constant  Value=MWS.In.VAFNMan(1)
  Constant3 : Constant  Value=MWS.In.VAFNManEn
  Constant4 : Constant  Value=MWS.In.EnLimitStop_VAFN  VectorParams1D=off
  Divide : Product  Inputs=**
  Multiport Switch : MultiPortSwitch  Inputs=4
  Mux2 : Mux  Inputs=2
  Switch1 : Switch  Criteria=u2 > Threshold
  VAFN FanRL Error Term : Subsystem
  VAFN Max Error Term : Subsystem
  VAFN Min Error Term : Subsystem
  VAFN Sched Error Term : Subsystem
  VAFN_Er : Outport
  LimVio : Outport  Port=2
  wires:
  Multiport Switch/1 -> Switch1/3
  VAFN Sched Error Term/1(VAFNEr) -> Multiport Switch/5  "VAFN schedule"
  Constant3/1 -> Switch1/2  "Enable Manual VAFN"
  Constant2/1 -> Switch1/1  "Manual VAFN"
  Switch1/1 -> VAFN_Er/1
  EngBus/1 -> [EngBus]
  InputBus/1 -> [InputBus]
  Constant1/1 -> Multiport Switch/1
  [EngBus] -> VAFN Sched Error Term/1(EngBus)
  [InputBus] -> VAFN Sched Error Term/2(InputBus)
  EngIndep/1 -> [EngIndep]
  VAFN Min Error Term/1(Er) -> Multiport Switch/3  "VAFN Min"
  VAFN Max Error Term/1(Er) -> Multiport Switch/4  "VAFN Max"
  VAFN Max Error Term/2(LimVio) -> [LV_VAFNMaxEr]
  VAFN Min Error Term/2(LimVio) -> [LV_VAFNMinEr]
  [InputBus] -> VAFN Max Error Term/1(InputBus), VAFN Min Error Term/1(InputBus)
  [EngBus] -> VAFN FanRL Error Term/1(EngBus)
  [EngIndep] -> VAFN FanRL Error Term/2(EngIndep)
  VAFN FanRL Error Term/1(Fan RLine) -> Multiport Switch/2
  Constant4/1 -> Divide/1
  [LV_VAFNMinEr] -> Mux2/1
  [LV_VAFNMaxEr] -> Mux2/2
  Mux2/1 -> Divide/2
  Divide/1 -> LimVio/1

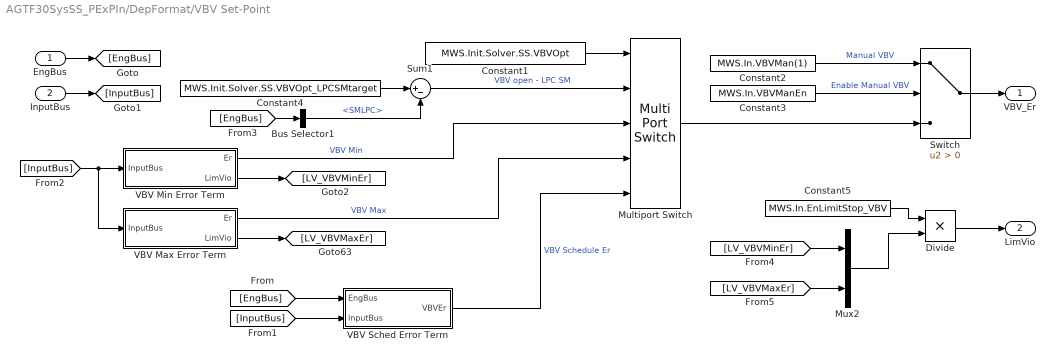
== system AGTF30SysSS_PExPIn/DepFormat/VBV Set-Point ==
  EngBus : Inport
  InputBus : Inport  Port=2
  Bus Selector1 : BusSelector  OutputSignals=SM.SMLPC
  Constant1 : Constant  Value=MWS.Init.Solver.SS.VBVOpt
  Constant2 : Constant  Value=MWS.In.VBVMan(1)
  Constant3 : Constant  Value=MWS.In.VBVManEn
  Constant4 : Constant  Value=MWS.Init.Solver.SS.VBVOpt_LPCSMtarget
  Constant5 : Constant  Value=MWS.In.EnLimitStop_VBV  VectorParams1D=off
  Divide : Product  Inputs=**
  Multiport Switch : MultiPortSwitch  Inputs=4
  Mux2 : Mux  Inputs=2
  Sum1 : Sum  Inputs=|+-
  Switch : Switch  Criteria=u2 > Threshold
  VBV Max Error Term : Subsystem
  VBV Min Error Term : Subsystem
  VBV Sched Error Term : Subsystem
  VBV_Er : Outport
  LimVio : Outport  Port=2
  wires:
  VBV Sched Error Term/1(VBVEr) -> Multiport Switch/5  "VBV Schedule Er"
  [InputBus] -> VBV Sched Error Term/2(InputBus)
  Sum1/1 -> Multiport Switch/2  "VBV open - LPC SM"
  Multiport Switch/1 -> Switch/3
  Switch/1 -> VBV_Er/1
  Constant2/1 -> Switch/1  "Manual VBV"
  Constant1/1 -> Multiport Switch/1
  Constant3/1 -> Switch/2  "Enable Manual VBV"
  InputBus/1 -> [InputBus]
  EngBus/1 -> [EngBus]
  [EngBus] -> VBV Sched Error Term/1(EngBus)
  [InputBus] -> VBV Max Error Term/1(InputBus), VBV Min Error Term/1(InputBus)
  Constant4/1 -> Sum1/1
  [EngBus] -> Bus Selector1/1
  Bus Selector1/1 -> Sum1/2  "<SMLPC>"
  VBV Max Error Term/2(LimVio) -> [LV_VBVMaxEr]
  VBV Min Error Term/2(LimVio) -> [LV_VBVMinEr]
  VBV Min Error Term/1(Er) -> Multiport Switch/3  "VBV Min"
  VBV Max Error Term/1(Er) -> Multiport Switch/4  "VBV Max"
  Mux2/1 -> Divide/2
  Constant5/1 -> Divide/1
  Divide/1 -> LimVio/1
  [LV_VBVMinEr] -> Mux2/1
  [LV_VBVMaxEr] -> Mux2/2

== system AGTF30SysSS_PExPIn/DepFormat/PInHPS Set-Point/PInHPS Sched Error Term ==
  EngBus : Inport
  InputBus : Inport  Port=2
  Bus Selector1 : BusSelector  OutputSignals=Shaft.N_HPC
  Bus Selector2 : BusSelector  OutputSignals=TrqInHPS
  Constant : Constant  Value=0
  Divide : Product  Inputs=**
  Gain : Gain  Gain=1/5252.113
  Sum : Sum  Inputs=|+-
  Terminator : Terminator
  Terminator1 : Terminator
  PInHPSEr : Outport
  wires:
  Bus Selector2/1 -> Divide/2  "<TrqInHPS>"
  InputBus/1 -> Terminator1/1, Bus Selector2/1
  Sum/1 -> PInHPSEr/1
  Constant/1 -> Sum/1
  EngBus/1 -> Bus Selector1/1, Terminator/1
  Bus Selector1/1 -> Divide/1  "<N_HPC>"
  Divide/1 -> Gain/1
  Gain/1 -> Sum/2

== system AGTF30SysSS_PExPIn/DepFormat/PInLPS Set-Point/PInLPS Sched Error Term ==
  EngBus : Inport
  InputBus : Inport  Port=2
  Bus Selector1 : BusSelector  OutputSignals=Shaft.N_LPC
  Bus Selector2 : BusSelector  OutputSignals=TrqInLPS
  Constant : Constant  Value=0
  Divide : Product  Inputs=**
  Gain : Gain  Gain=1/5252.113
  Sum : Sum  Inputs=|+-
  Terminator : Terminator
  Terminator1 : Terminator
  PInLPSEr : Outport
  wires:
  Bus Selector2/1 -> Divide/2  "<TrqInLPS>"
  InputBus/1 -> Terminator1/1, Bus Selector2/1
  Sum/1 -> PInLPSEr/1
  Constant/1 -> Sum/1
  EngBus/1 -> Bus Selector1/1, Terminator/1
  Bus Selector1/1 -> Divide/1  "<N_LPC>"
  Divide/1 -> Gain/1
  Gain/1 -> Sum/2

== system AGTF30SysSS_PExPIn/DepFormat/Primary Set-Point/Corrected Fan Speed Error Term ==
  note: Error in corrected speed vs Set Point
  EngBus : Inport
  InputBus : Inport  Port=2
  Bus Selector : BusSelector  OutputSignals=Data.FAN_Data.Nc
  Nc1 Sched Error Term : Subsystem
  Nc1 Set Point : Constant  Value=MWS.In.N1cMan(1)
  Nc1 Set Point1 : Constant  Value=MWS.In.N1cManEn
  Sum1 : Sum  Inputs=|+-
  Switch : Switch  Criteria=u2 > Threshold
  NcEr : Outport
  wires:
  Nc1 Set Point/1 -> Switch/1
  Bus Selector/1 -> Sum1/1  "<Nc>"
  EngBus/1 -> Bus Selector/1, Nc1 Sched Error Term/1(EngBus)
  Sum1/1 -> NcEr/1  "NcEr"
  InputBus/1 -> Nc1 Sched Error Term/2(InputBus)
  Nc1 Sched Error Term/1(Nc1Er) -> Switch/3  "N1c Schedule Er"
  Nc1 Set Point1/1 -> Switch/2
  Switch/1 -> Sum1/2

== system AGTF30SysSS_PExPIn/DepFormat/Primary Set-Point/Corrected Map Fan Speed Error Term ==
  note: Error in corrected speed vs Set Point
  EngBus : Inport
  Bus Selector : BusSelector  OutputSignals=Data.FAN_Data.NcMap
  N1c Map Set Point : Constant  Value=MWS.Init.Solver.Targets.N1cMap
  Sum1 : Sum  Inputs=|+-
  NcEr : Outport
  wires:
  N1c Map Set Point/1 -> Sum1/2
  Sum1/1 -> NcEr/1  "NcEr"
  EngBus/1 -> Bus Selector/1
  Bus Selector/1 -> Sum1/1  "<NcMap>"

== system AGTF30SysSS_PExPIn/DepFormat/Primary Set-Point/FAR Min Error Term ==
  EngBus : Inport
  Bus Selector : BusSelector  OutputSignals=S36.FAR
  Compare To Constant1 : simulink/Logic and Bit Operations/Compare To Constant  relop=~=  const=10  OutDataTypeStr=boolean
  Compare To Zero : simulink/Logic and Bit Operations/Compare To Zero  relop=<  OutDataTypeStr=boolean
      link override Compare: Operator=<  OutDataTypeStr=boolean
  Constant : Constant  Value=MWS.Init.Solver.Limits.FAR_Min
  Constant1 : Constant  Value=MWS.Init.Solver.Targets.Opt
  Logical Operator : Logic  AllPortsSameDT=off  OutDataTypeStr=boolean
  Sum1 : Sum  Inputs=|+-
  Er : Outport
  LimVio : Outport  Port=2
  wires:
  Sum1/1 -> Compare To Zero/1, Er/1
  EngBus/1 -> Bus Selector/1
  Bus Selector/1 -> Sum1/1  "<FAR>"
  Constant/1 -> Sum1/2
  Constant1/1 -> Compare To Constant1/1
  Compare To Constant1/1 -> Logical Operator/1
  Compare To Zero/1 -> Logical Operator/2
  Logical Operator/1 -> LimVio/1

== system AGTF30SysSS_PExPIn/DepFormat/Primary Set-Point/FanNcMap Max Error Term ==
  EngBus : Inport
  Bus Selector : BusSelector  OutputSignals=Data.FAN_Data.NcMap
  Compare To Constant1 : simulink/Logic and Bit Operations/Compare To Constant  relop=~=  const=15  OutDataTypeStr=boolean
  Compare To Zero : simulink/Logic and Bit Operations/Compare To Zero  relop=>  OutDataTypeStr=boolean
      link override Compare: Operator=>  OutDataTypeStr=boolean
  Constant : Constant  Value=MWS.Init.Solver.Limits.FanNcMap_Max
  Constant1 : Constant  Value=MWS.Init.Solver.Targets.Opt
  Logical Operator : Logic  AllPortsSameDT=off  OutDataTypeStr=boolean
  Sum1 : Sum  Inputs=|+-
  Er : Outport
  LimVio : Outport  Port=2
  wires:
  Logical Operator/1 -> LimVio/1
  Compare To Zero/1 -> Logical Operator/2
  Compare To Constant1/1 -> Logical Operator/1
  Constant1/1 -> Compare To Constant1/1
  Constant/1 -> Sum1/2
  Bus Selector/1 -> Sum1/1  "<NcMap>"
  EngBus/1 -> Bus Selector/1
  Sum1/1 -> Er/1, Compare To Zero/1

== system AGTF30SysSS_PExPIn/DepFormat/Primary Set-Point/FanNcMap Min Error Term ==
  EngBus : Inport
  Bus Selector : BusSelector  OutputSignals=Data.FAN_Data.NcMap
  Compare To Constant1 : simulink/Logic and Bit Operations/Compare To Constant  relop=~=  const=14  OutDataTypeStr=boolean
  Compare To Zero : simulink/Logic and Bit Operations/Compare To Zero  relop=<  OutDataTypeStr=boolean
      link override Compare: Operator=<  OutDataTypeStr=boolean
  Constant : Constant  Value=MWS.Init.Solver.Limits.FanNcMap_Min
  Constant1 : Constant  Value=MWS.Init.Solver.Targets.Opt
  Logical Operator : Logic  AllPortsSameDT=off  OutDataTypeStr=boolean
  Sum1 : Sum  Inputs=|+-
  Er : Outport
  LimVio : Outport  Port=2
  wires:
  Sum1/1 -> Compare To Zero/1, Er/1
  EngBus/1 -> Bus Selector/1
  Bus Selector/1 -> Sum1/1  "<NcMap>"
  Constant/1 -> Sum1/2
  Constant1/1 -> Compare To Constant1/1
  Compare To Constant1/1 -> Logical Operator/1
  Compare To Zero/1 -> Logical Operator/2
  Logical Operator/1 -> LimVio/1

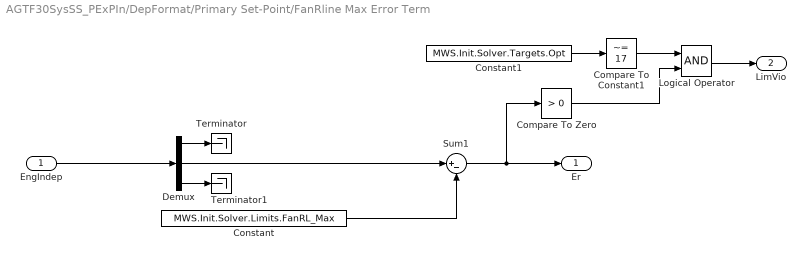
== system AGTF30SysSS_PExPIn/DepFormat/Primary Set-Point/FanRline Max Error Term ==
  EngIndep : Inport
  Compare To Constant1 : simulink/Logic and Bit Operations/Compare To Constant  relop=~=  const=17  OutDataTypeStr=boolean
  Compare To Zero : simulink/Logic and Bit Operations/Compare To Zero  relop=>  OutDataTypeStr=boolean
      link override Compare: Operator=>  OutDataTypeStr=boolean
  Constant : Constant  Value=MWS.Init.Solver.Limits.FanRL_Max
  Constant1 : Constant  Value=MWS.Init.Solver.Targets.Opt
  Demux : Demux  Outputs=[3 1 3]
  Logical Operator : Logic  AllPortsSameDT=off  OutDataTypeStr=boolean
  Sum1 : Sum  Inputs=|+-
  Terminator : Terminator
  Terminator1 : Terminator
  Er : Outport
  LimVio : Outport  Port=2
  wires:
  Demux/3 -> Terminator1/1
  Demux/1 -> Terminator/1
  Sum1/1 -> Compare To Zero/1, Er/1
  EngIndep/1 -> Demux/1
  Demux/2 -> Sum1/1
  Constant/1 -> Sum1/2
  Constant1/1 -> Compare To Constant1/1
  Compare To Constant1/1 -> Logical Operator/1
  Compare To Zero/1 -> Logical Operator/2
  Logical Operator/1 -> LimVio/1

== system AGTF30SysSS_PExPIn/DepFormat/Primary Set-Point/FanRline Min Error Term ==
  EngIndep : Inport
  Compare To Constant1 : simulink/Logic and Bit Operations/Compare To Constant  relop=~=  const=16  OutDataTypeStr=boolean
  Compare To Zero : simulink/Logic and Bit Operations/Compare To Zero  relop=<  OutDataTypeStr=boolean
      link override Compare: Operator=<  OutDataTypeStr=boolean
  Constant : Constant  Value=MWS.Init.Solver.Limits.FanRL_Min
  Constant1 : Constant  Value=MWS.Init.Solver.Targets.Opt
  Demux : Demux  Outputs=[3 1 3]
  Logical Operator : Logic  AllPortsSameDT=off  OutDataTypeStr=boolean
  Sum1 : Sum  Inputs=|+-
  Terminator : Terminator
  Terminator1 : Terminator
  Er : Outport
  LimVio : Outport  Port=2
  wires:
  Logical Operator/1 -> LimVio/1
  Compare To Zero/1 -> Logical Operator/2
  Compare To Constant1/1 -> Logical Operator/1
  Constant1/1 -> Compare To Constant1/1
  Constant/1 -> Sum1/2
  Demux/2 -> Sum1/1
  EngIndep/1 -> Demux/1
  Sum1/1 -> Er/1, Compare To Zero/1
  Demux/1 -> Terminator/1
  Demux/3 -> Terminator1/1

== system AGTF30SysSS_PExPIn/DepFormat/Primary Set-Point/FanSM Min Error Term ==
  EngBus : Inport
  Bus Selector : BusSelector  OutputSignals=SM.SMFan
  Compare To Constant1 : simulink/Logic and Bit Operations/Compare To Constant  relop=~=  const=11  OutDataTypeStr=boolean
  Compare To Zero : simulink/Logic and Bit Operations/Compare To Zero  relop=<  OutDataTypeStr=boolean
      link override Compare: Operator=<  OutDataTypeStr=boolean
  Constant : Constant  Value=MWS.Init.Solver.Limits.FanSM_Min
  Constant1 : Constant  Value=MWS.Init.Solver.Targets.Opt
  Logical Operator : Logic  AllPortsSameDT=off  OutDataTypeStr=boolean
  Sum1 : Sum  Inputs=|+-
  Er : Outport
  LimVio : Outport  Port=2
  wires:
  Logical Operator/1 -> LimVio/1
  Compare To Zero/1 -> Logical Operator/2
  Compare To Constant1/1 -> Logical Operator/1
  Constant1/1 -> Compare To Constant1/1
  Constant/1 -> Sum1/2
  Bus Selector/1 -> Sum1/1  "<SMFan>"
  EngBus/1 -> Bus Selector/1
  Sum1/1 -> Er/1, Compare To Zero/1

== system AGTF30SysSS_PExPIn/DepFormat/Primary Set-Point/HPCNcMap Max Error Term ==
  EngBus : Inport
  Bus Selector : BusSelector  OutputSignals=Data.HPC_Data.NcMap
  Compare To Constant1 : simulink/Logic and Bit Operations/Compare To Constant  relop=~=  const=23  OutDataTypeStr=boolean
  Compare To Zero : simulink/Logic and Bit Operations/Compare To Zero  relop=>  OutDataTypeStr=boolean
      link override Compare: Operator=>  OutDataTypeStr=boolean
  Constant : Constant  Value=MWS.Init.Solver.Limits.HPCNcMap_Max
  Constant1 : Constant  Value=MWS.Init.Solver.Targets.Opt
  Logical Operator : Logic  AllPortsSameDT=off  OutDataTypeStr=boolean
  Sum1 : Sum  Inputs=|+-
  Er : Outport
  LimVio : Outport  Port=2
  wires:
  Logical Operator/1 -> LimVio/1
  Compare To Zero/1 -> Logical Operator/2
  Compare To Constant1/1 -> Logical Operator/1
  Constant1/1 -> Compare To Constant1/1
  Constant/1 -> Sum1/2
  Bus Selector/1 -> Sum1/1  "<NcMap>"
  EngBus/1 -> Bus Selector/1
  Sum1/1 -> Er/1, Compare To Zero/1

== system AGTF30SysSS_PExPIn/DepFormat/Primary Set-Point/HPCNcMap Min Error Term ==
  EngBus : Inport
  Bus Selector : BusSelector  OutputSignals=Data.HPC_Data.NcMap
  Compare To Constant1 : simulink/Logic and Bit Operations/Compare To Constant  relop=~=  const=22  OutDataTypeStr=boolean
  Compare To Zero : simulink/Logic and Bit Operations/Compare To Zero  relop=<  OutDataTypeStr=boolean
      link override Compare: Operator=<  OutDataTypeStr=boolean
  Constant : Constant  Value=MWS.Init.Solver.Limits.HPCNcMap_Min
  Constant1 : Constant  Value=MWS.Init.Solver.Targets.Opt
  Logical Operator : Logic  AllPortsSameDT=off  OutDataTypeStr=boolean
  Sum1 : Sum  Inputs=|+-
  Er : Outport
  LimVio : Outport  Port=2
  wires:
  Sum1/1 -> Compare To Zero/1, Er/1
  EngBus/1 -> Bus Selector/1
  Bus Selector/1 -> Sum1/1  "<NcMap>"
  Constant/1 -> Sum1/2
  Constant1/1 -> Compare To Constant1/1
  Compare To Constant1/1 -> Logical Operator/1
  Compare To Zero/1 -> Logical Operator/2
  Logical Operator/1 -> LimVio/1

== system AGTF30SysSS_PExPIn/DepFormat/Primary Set-Point/HPCRline Max Error Term ==
  EngIndep : Inport
  Compare To Constant1 : simulink/Logic and Bit Operations/Compare To Constant  relop=~=  const=25  OutDataTypeStr=boolean
  Compare To Zero : simulink/Logic and Bit Operations/Compare To Zero  relop=>  OutDataTypeStr=boolean
      link override Compare: Operator=>  OutDataTypeStr=boolean
  Constant : Constant  Value=MWS.Init.Solver.Limits.HPCRL_Max
  Constant1 : Constant  Value=MWS.Init.Solver.Targets.Opt
  Demux : Demux  Outputs=[2 1 4]
  Logical Operator : Logic  AllPortsSameDT=off  OutDataTypeStr=boolean
  Sum1 : Sum  Inputs=|+-
  Terminator : Terminator
  Terminator1 : Terminator
  Er : Outport
  LimVio : Outport  Port=2
  wires:
  Demux/3 -> Terminator1/1
  Demux/1 -> Terminator/1
  Sum1/1 -> Compare To Zero/1, Er/1
  EngIndep/1 -> Demux/1
  Demux/2 -> Sum1/1
  Constant/1 -> Sum1/2
  Constant1/1 -> Compare To Constant1/1
  Compare To Constant1/1 -> Logical Operator/1
  Compare To Zero/1 -> Logical Operator/2
  Logical Operator/1 -> LimVio/1

== system AGTF30SysSS_PExPIn/DepFormat/Primary Set-Point/HPCRline Min Error Term ==
  EngIndep : Inport
  Compare To Constant1 : simulink/Logic and Bit Operations/Compare To Constant  relop=~=  const=24  OutDataTypeStr=boolean
  Compare To Zero : simulink/Logic and Bit Operations/Compare To Zero  relop=<  OutDataTypeStr=boolean
      link override Compare: Operator=<  OutDataTypeStr=boolean
  Constant : Constant  Value=MWS.Init.Solver.Limits.HPCRL_Min
  Constant1 : Constant  Value=MWS.Init.Solver.Targets.Opt
  Demux : Demux  Outputs=[2 1 4]
  Logical Operator : Logic  AllPortsSameDT=off  OutDataTypeStr=boolean
  Sum1 : Sum  Inputs=|+-
  Terminator : Terminator
  Terminator1 : Terminator
  Er : Outport
  LimVio : Outport  Port=2
  wires:
  Logical Operator/1 -> LimVio/1
  Compare To Zero/1 -> Logical Operator/2
  Compare To Constant1/1 -> Logical Operator/1
  Constant1/1 -> Compare To Constant1/1
  Constant/1 -> Sum1/2
  Demux/2 -> Sum1/1
  EngIndep/1 -> Demux/1
  Sum1/1 -> Er/1, Compare To Zero/1
  Demux/1 -> Terminator/1
  Demux/3 -> Terminator1/1

== system AGTF30SysSS_PExPIn/DepFormat/Primary Set-Point/HPCSM Min Error Term ==
  EngBus : Inport
  Bus Selector : BusSelector  OutputSignals=SM.SMHPC
  Compare To Constant1 : simulink/Logic and Bit Operations/Compare To Constant  relop=~=  const=13  OutDataTypeStr=boolean
  Compare To Zero : simulink/Logic and Bit Operations/Compare To Zero  relop=<  OutDataTypeStr=boolean
      link override Compare: Operator=<  OutDataTypeStr=boolean
  Constant : Constant  Value=MWS.Init.Solver.Limits.HPCSM_Min
  Constant1 : Constant  Value=MWS.Init.Solver.Targets.Opt
  Logical Operator : Logic  AllPortsSameDT=off  OutDataTypeStr=boolean
  Sum1 : Sum  Inputs=|+-
  Er : Outport
  LimVio : Outport  Port=2
  wires:
  Logical Operator/1 -> LimVio/1
  Compare To Zero/1 -> Logical Operator/2
  Compare To Constant1/1 -> Logical Operator/1
  Constant1/1 -> Compare To Constant1/1
  Constant/1 -> Sum1/2
  Bus Selector/1 -> Sum1/1  "<SMHPC>"
  EngBus/1 -> Bus Selector/1
  Sum1/1 -> Er/1, Compare To Zero/1

== system AGTF30SysSS_PExPIn/DepFormat/Primary Set-Point/HPTNcMap Max Error Term ==
  EngBus : Inport
  Bus Selector : BusSelector  OutputSignals=Data.HPT_Data.NcMap
  Compare To Constant1 : simulink/Logic and Bit Operations/Compare To Constant  relop=~=  const=27  OutDataTypeStr=boolean
  Compare To Zero : simulink/Logic and Bit Operations/Compare To Zero  relop=>  OutDataTypeStr=boolean
      link override Compare: Operator=>  OutDataTypeStr=boolean
  Constant : Constant  Value=MWS.Init.Solver.Limits.HPTNcMap_Max
  Constant1 : Constant  Value=MWS.Init.Solver.Targets.Opt
  Logical Operator : Logic  AllPortsSameDT=off  OutDataTypeStr=boolean
  Sum1 : Sum  Inputs=|+-
  Er : Outport
  LimVio : Outport  Port=2
  wires:
  Logical Operator/1 -> LimVio/1
  Compare To Zero/1 -> Logical Operator/2
  Compare To Constant1/1 -> Logical Operator/1
  Constant1/1 -> Compare To Constant1/1
  Constant/1 -> Sum1/2
  Bus Selector/1 -> Sum1/1  "<NcMap>"
  EngBus/1 -> Bus Selector/1
  Sum1/1 -> Er/1, Compare To Zero/1

== system AGTF30SysSS_PExPIn/DepFormat/Primary Set-Point/HPTNcMap Min Error Term ==
  EngBus : Inport
  Bus Selector : BusSelector  OutputSignals=Data.HPT_Data.NcMap
  Compare To Constant1 : simulink/Logic and Bit Operations/Compare To Constant  relop=~=  const=26  OutDataTypeStr=boolean
  Compare To Zero : simulink/Logic and Bit Operations/Compare To Zero  relop=<  OutDataTypeStr=boolean
      link override Compare: Operator=<  OutDataTypeStr=boolean
  Constant : Constant  Value=MWS.Init.Solver.Limits.HPTNcMap_Min
  Constant1 : Constant  Value=MWS.Init.Solver.Targets.Opt
  Logical Operator : Logic  AllPortsSameDT=off  OutDataTypeStr=boolean
  Sum1 : Sum  Inputs=|+-
  Er : Outport
  LimVio : Outport  Port=2
  wires:
  Sum1/1 -> Compare To Zero/1, Er/1
  EngBus/1 -> Bus Selector/1
  Bus Selector/1 -> Sum1/1  "<NcMap>"
  Constant/1 -> Sum1/2
  Constant1/1 -> Compare To Constant1/1
  Compare To Constant1/1 -> Logical Operator/1
  Compare To Zero/1 -> Logical Operator/2
  Logical Operator/1 -> LimVio/1

== system AGTF30SysSS_PExPIn/DepFormat/Primary Set-Point/HPTPRMap Max Error Term ==
  EngBus : Inport
  Bus Selector : BusSelector  OutputSignals=Data.HPT_Data.PRMap
  Compare To Constant1 : simulink/Logic and Bit Operations/Compare To Constant  relop=~=  const=29  OutDataTypeStr=boolean
  Compare To Zero : simulink/Logic and Bit Operations/Compare To Zero  relop=>  OutDataTypeStr=boolean
      link override Compare: Operator=>  OutDataTypeStr=boolean
  Constant : Constant  Value=MWS.Init.Solver.Limits.HPTPRMap_Max
  Constant1 : Constant  Value=MWS.Init.Solver.Targets.Opt
  Logical Operator : Logic  AllPortsSameDT=off  OutDataTypeStr=boolean
  Sum1 : Sum  Inputs=|+-
  Er : Outport
  LimVio : Outport  Port=2
  wires:
  Sum1/1 -> Compare To Zero/1, Er/1
  EngBus/1 -> Bus Selector/1
  Bus Selector/1 -> Sum1/1  "<PRMap>"
  Constant/1 -> Sum1/2
  Constant1/1 -> Compare To Constant1/1
  Compare To Constant1/1 -> Logical Operator/1
  Compare To Zero/1 -> Logical Operator/2
  Logical Operator/1 -> LimVio/1

== system AGTF30SysSS_PExPIn/DepFormat/Primary Set-Point/HPTPRMap Min Error Term ==
  EngBus : Inport
  Bus Selector : BusSelector  OutputSignals=Data.HPT_Data.PRMap
  Compare To Constant1 : simulink/Logic and Bit Operations/Compare To Constant  relop=~=  const=28  OutDataTypeStr=boolean
  Compare To Zero : simulink/Logic and Bit Operations/Compare To Zero  relop=<  OutDataTypeStr=boolean
      link override Compare: Operator=<  OutDataTypeStr=boolean
  Constant : Constant  Value=MWS.Init.Solver.Limits.HPTPRMap_Min
  Constant1 : Constant  Value=MWS.Init.Solver.Targets.Opt
  Logical Operator : Logic  AllPortsSameDT=off  OutDataTypeStr=boolean
  Sum1 : Sum  Inputs=|+-
  Er : Outport
  LimVio : Outport  Port=2
  wires:
  Logical Operator/1 -> LimVio/1
  Compare To Zero/1 -> Logical Operator/2
  Compare To Constant1/1 -> Logical Operator/1
  Constant1/1 -> Compare To Constant1/1
  Constant/1 -> Sum1/2
  Bus Selector/1 -> Sum1/1  "<PRMap>"
  EngBus/1 -> Bus Selector/1
  Sum1/1 -> Er/1, Compare To Zero/1

== system AGTF30SysSS_PExPIn/DepFormat/Primary Set-Point/LPCNcMap Max Error Term ==
  EngBus : Inport
  Bus Selector : BusSelector  OutputSignals=Data.LPC_Data.NcMap
  Compare To Constant1 : simulink/Logic and Bit Operations/Compare To Constant  relop=~=  const=19  OutDataTypeStr=boolean
  Compare To Zero : simulink/Logic and Bit Operations/Compare To Zero  relop=>  OutDataTypeStr=boolean
      link override Compare: Operator=>  OutDataTypeStr=boolean
  Constant : Constant  Value=MWS.Init.Solver.Limits.LPCNcMap_Max
  Constant1 : Constant  Value=MWS.Init.Solver.Targets.Opt
  Logical Operator : Logic  AllPortsSameDT=off  OutDataTypeStr=boolean
  Sum1 : Sum  Inputs=|+-
  Er : Outport
  LimVio : Outport  Port=2
  wires:
  Logical Operator/1 -> LimVio/1
  Compare To Zero/1 -> Logical Operator/2
  Compare To Constant1/1 -> Logical Operator/1
  Constant1/1 -> Compare To Constant1/1
  Constant/1 -> Sum1/2
  Bus Selector/1 -> Sum1/1  "<NcMap>"
  EngBus/1 -> Bus Selector/1
  Sum1/1 -> Er/1, Compare To Zero/1

== system AGTF30SysSS_PExPIn/DepFormat/Primary Set-Point/LPCNcMap Min Error Term ==
  EngBus : Inport
  Bus Selector : BusSelector  OutputSignals=Data.LPC_Data.NcMap
  Compare To Constant1 : simulink/Logic and Bit Operations/Compare To Constant  relop=~=  const=18  OutDataTypeStr=boolean
  Compare To Zero : simulink/Logic and Bit Operations/Compare To Zero  relop=<  OutDataTypeStr=boolean
      link override Compare: Operator=<  OutDataTypeStr=boolean
  Constant : Constant  Value=MWS.Init.Solver.Limits.LPCNcMap_Min
  Constant1 : Constant  Value=MWS.Init.Solver.Targets.Opt
  Logical Operator : Logic  AllPortsSameDT=off  OutDataTypeStr=boolean
  Sum1 : Sum  Inputs=|+-
  Er : Outport
  LimVio : Outport  Port=2
  wires:
  Sum1/1 -> Compare To Zero/1, Er/1
  EngBus/1 -> Bus Selector/1
  Bus Selector/1 -> Sum1/1  "<NcMap>"
  Constant/1 -> Sum1/2
  Constant1/1 -> Compare To Constant1/1
  Compare To Constant1/1 -> Logical Operator/1
  Compare To Zero/1 -> Logical Operator/2
  Logical Operator/1 -> LimVio/1
